simulink model "x220KVSSTN_slx"  (R2025a)
settings: Solver=VariableStepAuto  StartTime=0.0  StopTime=1  RelTol=1e-4
libraries: spsThreePhaseSeriesRLCLoadLib x16, spsThreePhasePISectionLineLib x15, spsThreePhaseBreakerLib x8, spsThreePhaseVIMeasurementLib x7, spsThreePhaseTransformerTwoWindingsLib x5, spsLoadFlowBusLib x4, spsThreePhaseSourceLib x3, spsRMSLib x1, spsThreePhaseFaultLib x1, sps_lib x1
settings Model: Creator=ARYAN CHOUDHARY  LastModifiedBy=ARYAN CHOUDHARY

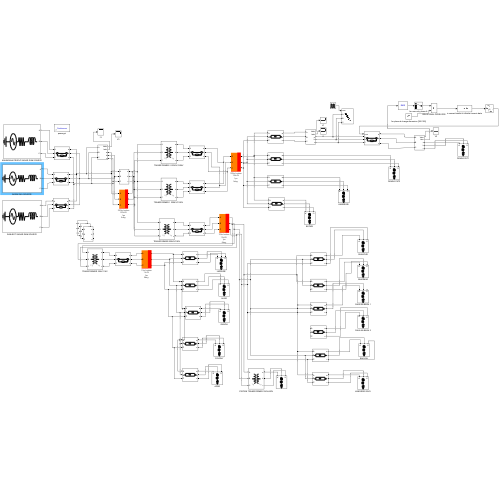
[thumbnail: Simulink's stored preview of the top-level diagram]
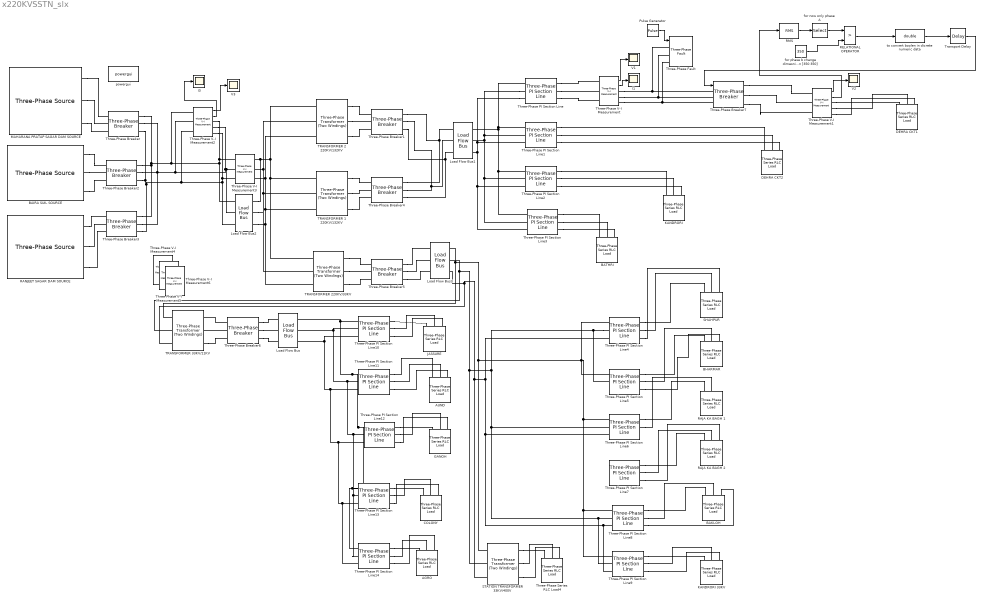
== system x220KVSSTN_slx ==
  AGRO : spsThreePhaseSeriesRLCLoadLib/Three-Phase Series RLC Load  LConnTagsString=A|B|C  Configuration=Y (grounded)  NominalVoltage=132e3  Vabc=[1e3 1e3 1e3]  Vabcp=[1e3 1e3 1e3]  NominalFrequency=50  UnbalancedPower=off  ActivePower=50e6  InductivePower=10e6  CapacitivePower=10e6  Pabc=[10e3 9e3 11e3]  QLabc=[100 90 110]  QCabc=[100 90 110]  Pabcp=[10e3 9e3 11e3]  QLabcp=[100 90 110]  QCabcp=[100 90 110]  Measurements=None  LoadType=constant PQ
  AUND : spsThreePhaseSeriesRLCLoadLib/Three-Phase Series RLC Load  LConnTagsString=A|B|C  Configuration=Y (grounded)  NominalVoltage=132e3  Vabc=[1e3 1e3 1e3]  Vabcp=[1e3 1e3 1e3]  NominalFrequency=50  UnbalancedPower=off  ActivePower=50e6  InductivePower=10e6  CapacitivePower=10e6  Pabc=[10e3 9e3 11e3]  QLabc=[100 90 110]  QCabc=[100 90 110]  Pabcp=[10e3 9e3 11e3]  QLabcp=[100 90 110]  QCabcp=[100 90 110]  Measurements=None  LoadType=constant PQ
  BAIRA SUIL SOURCE : spsThreePhaseSourceLib/Three-Phase Source  InternalConnection=Yg  VoltagePhases=off  Voltage=220e3  PhaseAngle=0  Voltage_phases=[25e3 25e3 25e3]/sqrt(3)  PhaseAngles_phases=[0 -120 +120]  Frequency=50  NonIdealSource=on  SpecifyImpedance=off  Resistance=0.8929  Inductance=16.58e-3  ShortCircuitLevel=100e6  BaseVoltage=25e3  XRratio=7  BusType=PQ  Pref=50e6  Qref=10e6  Prefabc=[10e3, 10e3, 10e3]  Qrefabc=[0, 0, 0]  Qmin=-inf  Qmax=inf
  BAKLOH : spsThreePhaseSeriesRLCLoadLib/Three-Phase Series RLC Load  LConnTagsString=A|B|C  Configuration=Y (grounded)  NominalVoltage=132e3  Vabc=[1e3 1e3 1e3]  Vabcp=[1e3 1e3 1e3]  NominalFrequency=50  UnbalancedPower=off  ActivePower=50e6  InductivePower=10e6  CapacitivePower=10e6  Pabc=[10e3 9e3 11e3]  QLabc=[100 90 110]  QCabc=[100 90 110]  Pabcp=[10e3 9e3 11e3]  QLabcp=[100 90 110]  QCabcp=[100 90 110]  Measurements=None  LoadType=constant PQ
  BATHRI : spsThreePhaseSeriesRLCLoadLib/Three-Phase Series RLC Load  LConnTagsString=A|B|C  Configuration=Y (grounded)  NominalVoltage=132e3  Vabc=[1e3 1e3 1e3]  Vabcp=[1e3 1e3 1e3]  NominalFrequency=50  UnbalancedPower=off  ActivePower=50e6  InductivePower=10e6  CapacitivePower=10e6  Pabc=[10e3 9e3 11e3]  QLabc=[100 90 110]  QCabc=[100 90 110]  Pabcp=[10e3 9e3 11e3]  QLabcp=[100 90 110]  QCabcp=[100 90 110]  Measurements=None  LoadType=constant PQ
  BHARMAR : spsThreePhaseSeriesRLCLoadLib/Three-Phase Series RLC Load  LConnTagsString=A|B|C  Configuration=Y (grounded)  NominalVoltage=132e3  Vabc=[1e3 1e3 1e3]  Vabcp=[1e3 1e3 1e3]  NominalFrequency=50  UnbalancedPower=off  ActivePower=50e6  InductivePower=10e6  CapacitivePower=10e6  Pabc=[10e3 9e3 11e3]  QLabc=[100 90 110]  QCabc=[100 90 110]  Pabcp=[10e3 9e3 11e3]  QLabcp=[100 90 110]  QCabcp=[100 90 110]  Measurements=None  LoadType=constant PQ
  COLONY : spsThreePhaseSeriesRLCLoadLib/Three-Phase Series RLC Load  LConnTagsString=A|B|C  Configuration=Y (grounded)  NominalVoltage=132e3  Vabc=[1e3 1e3 1e3]  Vabcp=[1e3 1e3 1e3]  NominalFrequency=50  UnbalancedPower=off  ActivePower=50e6  InductivePower=10e6  CapacitivePower=10e6  Pabc=[10e3 9e3 11e3]  QLabc=[100 90 110]  QCabc=[100 90 110]  Pabcp=[10e3 9e3 11e3]  QLabcp=[100 90 110]  QCabcp=[100 90 110]  Measurements=None  LoadType=constant PQ
  DEHRA CKT1 : spsThreePhaseSeriesRLCLoadLib/Three-Phase Series RLC Load  LConnTagsString=A|B|C  Configuration=Y (grounded)  NominalVoltage=132e3  Vabc=[1e3 1e3 1e3]  Vabcp=[1e3 1e3 1e3]  NominalFrequency=50  UnbalancedPower=off  ActivePower=50e6  InductivePower=10e6  CapacitivePower=10e6  Pabc=[10e3 9e3 11e3]  QLabc=[100 90 110]  QCabc=[100 90 110]  Pabcp=[10e3 9e3 11e3]  QLabcp=[100 90 110]  QCabcp=[100 90 110]  Measurements=None  LoadType=constant PQ
  DEHRA CKT2 : spsThreePhaseSeriesRLCLoadLib/Three-Phase Series RLC Load  LConnTagsString=A|B|C  Configuration=Y (grounded)  NominalVoltage=132e3  Vabc=[1e3 1e3 1e3]  Vabcp=[1e3 1e3 1e3]  NominalFrequency=50  UnbalancedPower=off  ActivePower=50e6  InductivePower=10e6  CapacitivePower=10e6  Pabc=[10e3 9e3 11e3]  QLabc=[100 90 110]  QCabc=[100 90 110]  Pabcp=[10e3 9e3 11e3]  QLabcp=[100 90 110]  QCabcp=[100 90 110]  Measurements=None  LoadType=constant PQ
  GANOH : spsThreePhaseSeriesRLCLoadLib/Three-Phase Series RLC Load  LConnTagsString=A|B|C  Configuration=Y (grounded)  NominalVoltage=132e3  Vabc=[1e3 1e3 1e3]  Vabcp=[1e3 1e3 1e3]  NominalFrequency=50  UnbalancedPower=off  ActivePower=50e6  InductivePower=10e6  CapacitivePower=10e6  Pabc=[10e3 9e3 11e3]  QLabc=[100 90 110]  QCabc=[100 90 110]  Pabcp=[10e3 9e3 11e3]  QLabcp=[100 90 110]  QCabcp=[100 90 110]  Measurements=None  LoadType=constant PQ
  I1 : Scope
      settings: ActiveDisplayYMinimum=-9501.2385556277131  ActiveDisplayYMaximum=13987.721223834153
  I3 : Scope
      settings: ActiveDisplayYMinimum=-31.371418582572904  ActiveDisplayYMaximum=38.377449294151894  DataLoggingVariableName=ScopeData4
  JASSURE : spsThreePhaseSeriesRLCLoadLib/Three-Phase Series RLC Load  LConnTagsString=A|B|C  Configuration=Y (grounded)  NominalVoltage=132e3  Vabc=[1e3 1e3 1e3]  Vabcp=[1e3 1e3 1e3]  NominalFrequency=50  UnbalancedPower=off  ActivePower=50e6  InductivePower=10e6  CapacitivePower=10e6  Pabc=[10e3 9e3 11e3]  QLabc=[100 90 110]  QCabc=[100 90 110]  Pabcp=[10e3 9e3 11e3]  QLabcp=[100 90 110]  QCabcp=[100 90 110]  Measurements=None  LoadType=constant PQ
  KANDRORI : spsThreePhaseSeriesRLCLoadLib/Three-Phase Series RLC Load  LConnTagsString=A|B|C  Configuration=Y (grounded)  NominalVoltage=132e3  Vabc=[1e3 1e3 1e3]  Vabcp=[1e3 1e3 1e3]  NominalFrequency=50  UnbalancedPower=off  ActivePower=50e6  InductivePower=10e6  CapacitivePower=10e6  Pabc=[10e3 9e3 11e3]  QLabc=[100 90 110]  QCabc=[100 90 110]  Pabcp=[10e3 9e3 11e3]  QLabcp=[100 90 110]  QCabcp=[100 90 110]  Measurements=None  LoadType=constant PQ
  KANDRORI 33KV : spsThreePhaseSeriesRLCLoadLib/Three-Phase Series RLC Load  LConnTagsString=A|B|C  Configuration=Y (grounded)  NominalVoltage=132e3  Vabc=[1e3 1e3 1e3]  Vabcp=[1e3 1e3 1e3]  NominalFrequency=50  UnbalancedPower=off  ActivePower=50e6  InductivePower=10e6  CapacitivePower=10e6  Pabc=[10e3 9e3 11e3]  QLabc=[100 90 110]  QCabc=[100 90 110]  Pabcp=[10e3 9e3 11e3]  QLabcp=[100 90 110]  QCabcp=[100 90 110]  Measurements=None  LoadType=constant PQ
  Load Flow Bus : spsLoadFlowBusLib/Load Flow Bus  LConnTagsString=a|b|c  RConnTagsString=a|b|c  Phases=ABC  Connectors=on both sides  ID=11kv busbar  Vbase=11e3  Vref=[1 1 1]  Vangle=[0 0 0]  VLF=1  VLFb=1  VLFc=1  angleLF=0  angleLFb=0  angleLFc=0
  Load Flow Bus1 : spsLoadFlowBusLib/Load Flow Bus  LConnTagsString=a|b|c  RConnTagsString=a|b|c  Phases=ABC  Connectors=on both sides  ID=132kv busbar  Vbase=132e3  Vref=[1 1 1]  Vangle=[0 0 0]  VLF=1  VLFb=1  VLFc=1  angleLF=0  angleLFb=0  angleLFc=0
  Load Flow Bus2 : spsLoadFlowBusLib/Load Flow Bus  LConnTagsString=a|b|c  RConnTagsString=a|b|c  Phases=ABC  Connectors=on both sides  ID=220kv busbar  Vbase=220e3  Vref=[1 1 1]  Vangle=[0 0 0]  VLF=1  VLFb=1  VLFc=1  angleLF=0  angleLFb=0  angleLFc=0
  Load Flow Bus3 : spsLoadFlowBusLib/Load Flow Bus  LConnTagsString=a|b|c  RConnTagsString=a|b|c  Phases=ABC  Connectors=on both sides  ID=33kv busbar  Vbase=33e3  Vref=[1 1 1]  Vangle=[0 0 0]  VLF=1  VLFb=1  VLFc=1  angleLF=0  angleLFb=0  angleLFc=0
  MAHARANA PRATAP SAGAR DAM SOURCE : spsThreePhaseSourceLib/Three-Phase Source  InternalConnection=Yg  VoltagePhases=off  Voltage=220e3  PhaseAngle=0  Voltage_phases=[25e3 25e3 25e3]/sqrt(3)  PhaseAngles_phases=[0 -120 +120]  Frequency=50  NonIdealSource=on  SpecifyImpedance=off  Resistance=0.8929  Inductance=16.58e-3  ShortCircuitLevel=100e6  BaseVoltage=25e3  XRratio=7  BusType=swing  Pref=10e3  Qref=0  Prefabc=[10e3, 10e3, 10e3]  Qrefabc=[0, 0, 0]  Qmin=-inf  Qmax=inf
  Pulse Generator : DiscretePulseGenerator  PulseType=Time based  Period=10  PhaseDelay=0.2
  RAJA KA BAGH 1 : spsThreePhaseSeriesRLCLoadLib/Three-Phase Series RLC Load  LConnTagsString=A|B|C  Configuration=Y (grounded)  NominalVoltage=132e3  Vabc=[1e3 1e3 1e3]  Vabcp=[1e3 1e3 1e3]  NominalFrequency=50  UnbalancedPower=off  ActivePower=50e6  InductivePower=10e6  CapacitivePower=10e6  Pabc=[10e3 9e3 11e3]  QLabc=[100 90 110]  QCabc=[100 90 110]  Pabcp=[10e3 9e3 11e3]  QLabcp=[100 90 110]  QCabcp=[100 90 110]  Measurements=None  LoadType=constant PQ
  RAJA KA BAGH 2 : spsThreePhaseSeriesRLCLoadLib/Three-Phase Series RLC Load  LConnTagsString=A|B|C  Configuration=Y (grounded)  NominalVoltage=132e3  Vabc=[1e3 1e3 1e3]  Vabcp=[1e3 1e3 1e3]  NominalFrequency=50  UnbalancedPower=off  ActivePower=50e6  InductivePower=10e6  CapacitivePower=10e6  Pabc=[10e3 9e3 11e3]  QLabc=[100 90 110]  QCabc=[100 90 110]  Pabcp=[10e3 9e3 11e3]  QLabcp=[100 90 110]  QCabcp=[100 90 110]  Measurements=None  LoadType=constant PQ
  RANJEET SAGAR DAM SOURCE : spsThreePhaseSourceLib/Three-Phase Source  InternalConnection=Yg  VoltagePhases=off  Voltage=220e3  PhaseAngle=0  Voltage_phases=[25e3 25e3 25e3]/sqrt(3)  PhaseAngles_phases=[0 -120 +120]  Frequency=50  NonIdealSource=on  SpecifyImpedance=off  Resistance=0.8929  Inductance=16.58e-3  ShortCircuitLevel=100e6  BaseVoltage=25e3  XRratio=7  BusType=PQ  Pref=50e6  Qref=10e6  Prefabc=[10e3, 10e3, 10e3]  Qrefabc=[0, 0, 0]  Qmin=-inf  Qmax=inf
  RELATIONAL OPERATOR : RelationalOperator  Operator=>  OutDataTypeStr=boolean  RndMeth=Simplest  InputSameDT=off
  RMS : spsRMSLib/RMS  TrueRMS=on  Freq=50  RMSInit=341  Ts=0
  SHAHPUR : spsThreePhaseSeriesRLCLoadLib/Three-Phase Series RLC Load  LConnTagsString=A|B|C  Configuration=Y (grounded)  NominalVoltage=132e3  Vabc=[1e3 1e3 1e3]  Vabcp=[1e3 1e3 1e3]  NominalFrequency=50  UnbalancedPower=off  ActivePower=50e6  InductivePower=10e6  CapacitivePower=10e6  Pabc=[10e3 9e3 11e3]  QLabc=[100 90 110]  QCabc=[100 90 110]  Pabcp=[10e3 9e3 11e3]  QLabcp=[100 90 110]  QCabcp=[100 90 110]  Measurements=None  LoadType=constant PQ
  STATION TRANSFORMER 33KV/400V : spsThreePhaseTransformerTwoWindingsLib/Three-Phase Transformer (Two Windings)  Winding1Connection=Yg  Winding2Connection=Yg  CoreType=Three single-phase transformers  SetSaturation=off  Hysteresis=off  DataFile='hysteresis'  SetInitialFlux=off  Measurements=None  UNITS=pu  NominalPower=[ 400e3 , 50 ]  Winding1=[33e3 , 0.002 , 0.08 ]  Winding2=[4e2 , 0.002 , 0.08 ]  Rm=500  Lm=500  L0=0.5  Saturation=[ 0,0 ; 0.0024,1.2 ; 1.0,1.52 ]  InitialFluxes=[ 0.8 , -0.8 , 0.7 ]  BreakLoop=off  DiscreteSolver=Trapezoidal iterative  DataType=off  TransfoNumber=1
  "TRANSFORMER 1 220KV/132KV " : spsThreePhaseTransformerTwoWindingsLib/Three-Phase Transformer (Two Windings)  Winding1Connection=Yg  Winding2Connection=Yg  CoreType=Three single-phase transformers  SetSaturation=off  Hysteresis=off  DataFile='hysteresis'  SetInitialFlux=off  Measurements=None  UNITS=pu  NominalPower=[ 63e6 , 50 ]  Winding1=[ 220e3 , 0.002 , 0.08 ]  Winding2=[ 132e3 , 0.002 , 0.08 ]  Rm=500  Lm=500  L0=0.5  Saturation=[ 0,0 ; 0.0024,1.2 ; 1.0,1.52 ]  InitialFluxes=[ 0.8 , -0.8 , 0.7 ]  BreakLoop=off  DiscreteSolver=Trapezoidal iterative  DataType=off  TransfoNumber=1
  TRANSFORMER 2 220KV/132KV : spsThreePhaseTransformerTwoWindingsLib/Three-Phase Transformer (Two Windings)  Winding1Connection=Yg  Winding2Connection=Yg  CoreType=Three single-phase transformers  SetSaturation=off  Hysteresis=off  DataFile='hysteresis'  SetInitialFlux=off  Measurements=None  UNITS=pu  NominalPower=[ 150e6 , 50 ]  Winding1=[ 220e3 , 0.002 , 0.08 ]  Winding2=[ 132e3 , 0.002 , 0.08 ]  Rm=500  Lm=500  L0=0.5  Saturation=[ 0,0 ; 0.0024,1.2 ; 1.0,1.52 ]  InitialFluxes=[ 0.8 , -0.8 , 0.7 ]  BreakLoop=off  DiscreteSolver=Trapezoidal iterative  DataType=off  TransfoNumber=1
  TRANSFORMER 220KV/33KV : spsThreePhaseTransformerTwoWindingsLib/Three-Phase Transformer (Two Windings)  Winding1Connection=Yg  Winding2Connection=Yg  CoreType=Three single-phase transformers  SetSaturation=off  Hysteresis=off  DataFile='hysteresis'  SetInitialFlux=off  Measurements=None  UNITS=pu  NominalPower=[ 31.5e6 , 50 ]  Winding1=[ 220e3 , 0.002 , 0.08 ]  Winding2=[33e3 , 0.002 , 0.08 ]  Rm=500  Lm=500  L0=0.5  Saturation=[ 0,0 ; 0.0024,1.2 ; 1.0,1.52 ]  InitialFluxes=[ 0.8 , -0.8 , 0.7 ]  BreakLoop=off  DiscreteSolver=Trapezoidal iterative  DataType=off  TransfoNumber=1
  TRANSFORMER 33KV/11KV : spsThreePhaseTransformerTwoWindingsLib/Three-Phase Transformer (Two Windings)  Winding1Connection=Yg  Winding2Connection=Yg  CoreType=Three single-phase transformers  SetSaturation=off  Hysteresis=off  DataFile='hysteresis'  SetInitialFlux=off  Measurements=None  UNITS=pu  NominalPower=[ 10e6 , 50 ]  Winding1=[33e3 , 0.002 , 0.08 ]  Winding2=[11e3 , 0.002 , 0.08 ]  Rm=500  Lm=500  L0=0.5  Saturation=[ 0,0 ; 0.0024,1.2 ; 1.0,1.52 ]  InitialFluxes=[ 0.8 , -0.8 , 0.7 ]  BreakLoop=off  DiscreteSolver=Trapezoidal iterative  DataType=off  TransfoNumber=1
  Three-Phase PI Section Line : spsThreePhasePISectionLineLib/Three-Phase PI Section Line  LConnTagsString=a|b|c  RConnTagsString=A|B|C  Length=34  Frequency=50  Resistances=[ 0.01273 0.3864]  Inductances="[ 0.9337e-3  4.1264e-3]"  Capacitances=[12.74e-9 7.751e-9]
  Three-Phase PI Section Line{1..14} (14 alike) : spsThreePhasePISectionLineLib/Three-Phase PI Section Line  LConnTagsString=a|b|c  RConnTagsString=A|B|C  Length=100  Frequency=50  Resistances=[ 0.01273 0.3864]  Inductances="[ 0.9337e-3  4.1264e-3]"  Capacitances=[12.74e-9 7.751e-9]
  Three-Phase Series RLC Load4 : spsThreePhaseSeriesRLCLoadLib/Three-Phase Series RLC Load  LConnTagsString=A|B|C  Configuration=Y (grounded)  NominalVoltage=132e3  Vabc=[1e3 1e3 1e3]  Vabcp=[1e3 1e3 1e3]  NominalFrequency=50  UnbalancedPower=off  ActivePower=320e3  InductivePower=200e3  CapacitivePower=50e3  Pabc=[10e3 9e3 11e3]  QLabc=[100 90 110]  QCabc=[100 90 110]  Pabcp=[10e3 9e3 11e3]  QLabcp=[100 90 110]  QCabcp=[100 90 110]  Measurements=None  LoadType=constant Z
  Three-Phase V-I Measurement : spsThreePhaseVIMeasurementLib/Three-Phase V-I Measurement  VoltageMeasurement=phase-to-ground  SetLabelV=off  LabelV=Vabc  Vpu=off  VpuLL=off  CurrentMeasurement=yes  SetLabelI=off  LabelI=Iabc  Ipu=off  Pbase=100e6  Vbase=500e3  OutputType=Complex  PhasorSimulation=off  PSBequivalent=0
  Three-Phase V-I Measurement1 : spsThreePhaseVIMeasurementLib/Three-Phase V-I Measurement  VoltageMeasurement=phase-to-ground  SetLabelV=off  LabelV=Vabc  Vpu=off  VpuLL=off  CurrentMeasurement=yes  SetLabelI=off  LabelI=Iabc  Ipu=off  Pbase=100e6  Vbase=500e3  OutputType=Complex  PhasorSimulation=off  PSBequivalent=0
  Three-Phase V-I Measurement2 : spsThreePhaseVIMeasurementLib/Three-Phase V-I Measurement  VoltageMeasurement=phase-to-ground  SetLabelV=off  LabelV=Vabc  Vpu=off  VpuLL=off  CurrentMeasurement=yes  SetLabelI=off  LabelI=Iabc  Ipu=off  Pbase=100e6  Vbase=500e3  OutputType=Complex  PhasorSimulation=off  PSBequivalent=0
  Three-Phase V-I Measurement{3..6} (4 alike) : spsThreePhaseVIMeasurementLib/Three-Phase V-I Measurement  VoltageMeasurement=no  SetLabelV=off  LabelV=Vabc  Vpu=off  VpuLL=off  CurrentMeasurement=no  SetLabelI=off  LabelI=Iabc  Ipu=off  Pbase=100e6  Vbase=500e3  OutputType=Complex  PhasorSimulation=off  PSBequivalent=0
  Three-Phase Breaker{,1..6} (7 alike) : spsThreePhaseBreakerLib/Three-Phase Breaker  InitialState=closed  SwitchA=on  SwitchB=on  SwitchC=on  SwitchTimes="[1/60  5/60]"  External=off  BreakerResistance=0.11  SnubberResistance=1e6  SnubberCapacitance=inf  Measurements=None
  Three-Phase Breaker7 : spsThreePhaseBreakerLib/Three-Phase Breaker  InitialState=closed  SwitchA=on  SwitchB=on  SwitchC=on  SwitchTimes="[1/60  5/60]"  External=on  BreakerResistance=0.11  SnubberResistance=1e6  SnubberCapacitance=inf  Measurements=None
  Three-Phase Fault : spsThreePhaseFaultLib/Three-Phase Fault  InitialStates=0  FaultA=on  FaultB=off  FaultC=off  GroundFault=on  SwitchTimes="[1/60  5/60]"  External=on  SwitchStatus=NaN  FaultResistance=0.01  GroundResistance=0.01  SnubberResistance=1e6  SnubberCapacitance=inf  Measurements=None
  Transport Delay : TransportDelay  DelayTime=0.2  BufferSize=30720
  V1 : Scope
      settings: ActiveDisplayYMinimum=-134175.28868127437  ActiveDisplayYMaximum=134108.09321994495
  V2 : Scope
      settings: ActiveDisplayYMinimum=-26718.305240557729  ActiveDisplayYMaximum=43984.791474851641  DataLoggingVariableName=ScopeData2
  V3 : Scope
      settings: ActiveDisplayYMinimum=-102465.81313536782  ActiveDisplayYMaximum=252772.60043735284  DataLoggingVariableName=ScopeData5
  for now only phase A : Selector  InputPortWidth=3  IndexOptions=Index vector (dialog)  Indices=1  OutputSizes=1
  for phase b change dimesnion [350 350] : Constant  Value=350  VectorParams1D=off
  powergui : sps_lib/powergui  Priority=1  SimulationMode=Continuous  SampleTime=50e-6  frequency=50  Iterations=50  frequencyindice=50  Pbase=100e6  ErrMax=1e-4  UnitsV=kV  UnitsW=MW  buscounter=0  FunctionMessages=off  echomessages=off  EnableUseOfTLC=off  CurrentSourceSwitches=off  DisableSnubberDevices=off  DisableRonSwitches=off  DisableVfSwitches=off  DisplayEquations=off  AutomaticDiscreteSolvers=off  SolverType=Tustin/Backward Euler (TBE)  Interpol=off  ExternalGateDelay=off  methode=off  Ts=100  x0status=blocks  SPID=on  SwTol=0  HookPort=off  NonlinearTolerance=1e-4  nMaxIteration=100  ContinueOnMaxIteration=off  RestoreLinks=warning  ResistiveCurrentMeasurement=off  Frange=[0:2:500]  Ylog=off  Xlog=on  ShowGrid=off  save=off  variable=ZData  structure=0  ZoomFFT=off  StartTime=0.0  cycles=1  DisplayStyle=1  fundamental=60  FreqAxis=off  MaxFrequency=1000  frequencyindicesteady=1  RmsSteady=1  display=off
  "to convert boolen in dicrete numeric data " : DataTypeConversion  OutDataTypeStr=double  SaturateOnIntegerOverflow=off  RndMeth=Floor
  wires:
  Three-Phase V-I Measurement/1 -> V1/1
  Three-Phase V-I Measurement/2 -> I1/1
  Three-Phase V-I Measurement1/1 -> V2/1
  Three-Phase V-I Measurement1/2 -> RMS/1
  Three-Phase V-I Measurement2/1 -> V3/1
  Three-Phase V-I Measurement2/2 -> I3/1
  Pulse Generator/1 -> Three-Phase Fault/1
  RELATIONAL OPERATOR/1 -> "to convert boolen in dicrete numeric data "/1
  Transport Delay/1 -> Three-Phase Breaker7/1
  RMS/1 -> for now only phase A/1
  for now only phase A/1 -> RELATIONAL OPERATOR/1
  for phase b change dimesnion [350 350]/1 -> RELATIONAL OPERATOR/2
  "to convert boolen in dicrete numeric data "/1 -> Transport Delay/1
  connections:
  MAHARANA PRATAP SAGAR DAM SOURCE/RConn1 -- Three-Phase Breaker/LConn1
  MAHARANA PRATAP SAGAR DAM SOURCE/RConn2 -- Three-Phase Breaker/LConn2
  MAHARANA PRATAP SAGAR DAM SOURCE/RConn3 -- Three-Phase Breaker/LConn3
  TRANSFORMER 2 220KV/132KV/RConn1 -- Three-Phase Breaker1/LConn1
  TRANSFORMER 2 220KV/132KV/RConn2 -- Three-Phase Breaker1/LConn2
  TRANSFORMER 2 220KV/132KV/RConn3 -- Three-Phase Breaker1/LConn3
  BAIRA SUIL SOURCE/RConn1 -- Three-Phase Breaker2/LConn1
  BAIRA SUIL SOURCE/RConn2 -- Three-Phase Breaker2/LConn2
  BAIRA SUIL SOURCE/RConn3 -- Three-Phase Breaker2/LConn3
  RANJEET SAGAR DAM SOURCE/RConn1 -- Three-Phase Breaker3/LConn1
  RANJEET SAGAR DAM SOURCE/RConn2 -- Three-Phase Breaker3/LConn2
  RANJEET SAGAR DAM SOURCE/RConn3 -- Three-Phase Breaker3/LConn3
  Three-Phase Breaker/RConn1 -- Three-Phase Breaker3/RConn1 -- Three-Phase Breaker2/RConn1 -- Three-Phase V-I Measurement2/LConn1 -- Three-Phase V-I Measurement3/LConn1 -- Three-Phase V-I Measurement2/RConn1 -- Load Flow Bus2/LConn1
  Three-Phase Breaker2/RConn2 -- Three-Phase Breaker3/RConn2 -- Three-Phase Breaker/RConn2 -- Three-Phase V-I Measurement2/LConn2 -- Load Flow Bus2/LConn2 -- Three-Phase V-I Measurement3/LConn2 -- Three-Phase V-I Measurement2/RConn2
  Three-Phase Breaker/RConn3 -- Three-Phase Breaker3/RConn3 -- Three-Phase V-I Measurement2/LConn3 -- Load Flow Bus2/LConn3 -- Three-Phase V-I Measurement2/RConn3 -- Three-Phase V-I Measurement3/LConn3 -- Three-Phase Breaker2/RConn3
  TRANSFORMER 220KV/33KV/LConn1 -- "TRANSFORMER 1 220KV/132KV "/LConn1 -- TRANSFORMER 2 220KV/132KV/LConn1 -- Load Flow Bus2/RConn1 -- Three-Phase V-I Measurement3/RConn1
  "TRANSFORMER 1 220KV/132KV "/LConn2 -- TRANSFORMER 220KV/33KV/LConn2 -- Load Flow Bus2/RConn2 -- Three-Phase V-I Measurement3/RConn2 -- TRANSFORMER 2 220KV/132KV/LConn2
  "TRANSFORMER 1 220KV/132KV "/LConn3 -- Load Flow Bus2/RConn3 -- TRANSFORMER 220KV/33KV/LConn3 -- Three-Phase V-I Measurement3/RConn3 -- TRANSFORMER 2 220KV/132KV/LConn3
  "TRANSFORMER 1 220KV/132KV "/RConn1 -- Three-Phase Breaker4/LConn1
  "TRANSFORMER 1 220KV/132KV "/RConn2 -- Three-Phase Breaker4/LConn2
  "TRANSFORMER 1 220KV/132KV "/RConn3 -- Three-Phase Breaker4/LConn3
  Three-Phase Breaker1/RConn1 -- Three-Phase Breaker4/RConn1 -- Load Flow Bus1/LConn1
  Three-Phase Breaker1/RConn2 -- Three-Phase Breaker4/RConn2 -- Load Flow Bus1/LConn2
  Three-Phase Breaker1/RConn3 -- Three-Phase Breaker4/RConn3 -- Load Flow Bus1/LConn3
  TRANSFORMER 220KV/33KV/RConn1 -- Three-Phase Breaker5/LConn1
  TRANSFORMER 220KV/33KV/RConn2 -- Three-Phase Breaker5/LConn2
  TRANSFORMER 220KV/33KV/RConn3 -- Three-Phase Breaker5/LConn3
  Three-Phase Breaker5/RConn1 -- Load Flow Bus3/LConn1
  Three-Phase Breaker5/RConn2 -- Load Flow Bus3/LConn2
  Three-Phase Breaker5/RConn3 -- Load Flow Bus3/LConn3
  Three-Phase PI Section Line/LConn1 -- Three-Phase PI Section Line3/LConn1 -- Three-Phase PI Section Line2/LConn1 -- Load Flow Bus1/RConn1 -- Three-Phase PI Section Line1/LConn1
  Three-Phase PI Section Line/LConn2 -- Three-Phase PI Section Line3/LConn2 -- Three-Phase PI Section Line2/LConn2 -- Load Flow Bus1/RConn2 -- Three-Phase PI Section Line1/LConn2
  Three-Phase PI Section Line/LConn3 -- Three-Phase PI Section Line3/LConn3 -- Three-Phase PI Section Line2/LConn3 -- Load Flow Bus1/RConn3 -- Three-Phase PI Section Line1/LConn3
  Three-Phase Fault/LConn1 -- Three-Phase V-I Measurement/RConn1 -- Three-Phase Breaker7/LConn1
  Three-Phase Fault/LConn2 -- Three-Phase V-I Measurement/RConn2 -- Three-Phase Breaker7/LConn2
  Three-Phase Fault/LConn3 -- Three-Phase V-I Measurement/RConn3 -- Three-Phase Breaker7/LConn3
  Three-Phase PI Section Line1/RConn1 -- DEHRA CKT2/LConn1
  Three-Phase PI Section Line1/RConn2 -- DEHRA CKT2/LConn2
  Three-Phase PI Section Line1/RConn3 -- DEHRA CKT2/LConn3
  Three-Phase PI Section Line2/RConn1 -- KANDRORI/LConn1
  Three-Phase PI Section Line2/RConn2 -- KANDRORI/LConn2
  Three-Phase PI Section Line2/RConn3 -- KANDRORI/LConn3
  Three-Phase PI Section Line3/RConn1 -- BATHRI/LConn1
  Three-Phase PI Section Line3/RConn2 -- BATHRI/LConn2
  Three-Phase PI Section Line3/RConn3 -- BATHRI/LConn3
  Three-Phase PI Section Line4/RConn1 -- SHAHPUR/LConn1
  Three-Phase PI Section Line4/RConn2 -- SHAHPUR/LConn2
  Three-Phase PI Section Line4/RConn3 -- SHAHPUR/LConn3
  Three-Phase PI Section Line5/RConn1 -- BHARMAR/LConn1
  Three-Phase PI Section Line5/RConn2 -- BHARMAR/LConn2
  Three-Phase PI Section Line5/RConn3 -- BHARMAR/LConn3
  Three-Phase PI Section Line6/RConn1 -- RAJA KA BAGH 1/LConn1
  Three-Phase PI Section Line6/RConn2 -- RAJA KA BAGH 1/LConn2
  Three-Phase PI Section Line7/RConn1 -- RAJA KA BAGH 2/LConn1
  Three-Phase PI Section Line7/RConn2 -- RAJA KA BAGH 2/LConn2
  Three-Phase PI Section Line7/RConn3 -- RAJA KA BAGH 2/LConn3
  Three-Phase PI Section Line8/RConn1 -- BAKLOH/LConn1
  Three-Phase PI Section Line8/RConn2 -- BAKLOH/LConn2
  Three-Phase PI Section Line8/RConn3 -- BAKLOH/LConn3
  Three-Phase PI Section Line9/RConn1 -- KANDRORI 33KV/LConn1
  Three-Phase PI Section Line9/RConn2 -- KANDRORI 33KV/LConn2
  Three-Phase PI Section Line9/RConn3 -- KANDRORI 33KV/LConn3
  Three-Phase PI Section Line4/LConn2 -- Load Flow Bus3/RConn2 -- TRANSFORMER 33KV/11KV/LConn2 -- STATION TRANSFORMER 33KV/400V/LConn2 -- Three-Phase PI Section Line8/LConn2 -- Three-Phase PI Section Line9/LConn2 -- Three-Phase PI Section Line6/LConn2 -- Three-Phase PI Section Line5/LConn2
  Three-Phase PI Section Line9/LConn3 -- Three-Phase PI Section Line6/LConn3 -- TRANSFORMER 33KV/11KV/LConn3 -- Load Flow Bus3/RConn3 -- STATION TRANSFORMER 33KV/400V/LConn3 -- Three-Phase PI Section Line4/LConn3 -- Three-Phase PI Section Line8/LConn3
  Three-Phase PI Section Line5/LConn1 -- Load Flow Bus3/RConn1 -- TRANSFORMER 33KV/11KV/LConn1 -- STATION TRANSFORMER 33KV/400V/LConn1 -- Three-Phase PI Section Line6/LConn1 -- Three-Phase PI Section Line9/LConn1 -- Three-Phase PI Section Line8/LConn1 -- Three-Phase PI Section Line4/LConn1
  STATION TRANSFORMER 33KV/400V/RConn1 -- Three-Phase Series RLC Load4/LConn1
  STATION TRANSFORMER 33KV/400V/RConn2 -- Three-Phase Series RLC Load4/LConn2
  STATION TRANSFORMER 33KV/400V/RConn3 -- Three-Phase Series RLC Load4/LConn3
  Three-Phase Breaker6/LConn1 -- TRANSFORMER 33KV/11KV/RConn1
  Three-Phase Breaker6/LConn2 -- TRANSFORMER 33KV/11KV/RConn2
  TRANSFORMER 33KV/11KV/RConn3 -- Three-Phase Breaker6/LConn3
  Three-Phase Breaker6/RConn1 -- Load Flow Bus/LConn1
  Three-Phase Breaker6/RConn2 -- Load Flow Bus/LConn2
  Three-Phase Breaker6/RConn3 -- Load Flow Bus/LConn3
  Three-Phase PI Section Line11/LConn1 -- Three-Phase PI Section Line14/LConn1 -- Three-Phase PI Section Line13/LConn1 -- Three-Phase PI Section Line12/LConn1 -- Three-Phase PI Section Line10/LConn1 -- Load Flow Bus/RConn1
  Three-Phase PI Section Line11/LConn2 -- Three-Phase PI Section Line14/LConn2 -- Three-Phase PI Section Line13/LConn2 -- Three-Phase PI Section Line12/LConn2 -- Three-Phase PI Section Line10/LConn2 -- Load Flow Bus/RConn2
  Three-Phase PI Section Line11/LConn3 -- Three-Phase PI Section Line13/LConn3 -- Three-Phase PI Section Line14/LConn3 -- Three-Phase PI Section Line12/LConn3 -- Three-Phase PI Section Line10/LConn3 -- Load Flow Bus/RConn3
  Three-Phase PI Section Line14/RConn1 -- AGRO/LConn1
  Three-Phase PI Section Line14/RConn2 -- AGRO/LConn2
  Three-Phase PI Section Line14/RConn3 -- AGRO/LConn3
  Three-Phase PI Section Line13/RConn1 -- COLONY/LConn1
  Three-Phase PI Section Line13/RConn2 -- COLONY/LConn2
  Three-Phase PI Section Line13/RConn3 -- COLONY/LConn3
  Three-Phase PI Section Line12/RConn1 -- GANOH/LConn1
  Three-Phase PI Section Line12/RConn2 -- GANOH/LConn2
  Three-Phase PI Section Line12/RConn3 -- GANOH/LConn3
  Three-Phase PI Section Line11/RConn1 -- AUND/LConn1
  Three-Phase PI Section Line11/RConn2 -- AUND/LConn2
  Three-Phase PI Section Line11/RConn3 -- AUND/LConn3
  Three-Phase PI Section Line10/RConn1 -- JASSURE/LConn1
  Three-Phase PI Section Line10/RConn2 -- JASSURE/LConn2
  Three-Phase PI Section Line10/RConn3 -- JASSURE/LConn3
  Three-Phase PI Section Line/RConn1 -- Three-Phase V-I Measurement/LConn1
  Three-Phase PI Section Line/RConn2 -- Three-Phase V-I Measurement/LConn2
  Three-Phase PI Section Line/RConn3 -- Three-Phase V-I Measurement/LConn3
  Three-Phase Breaker7/RConn1 -- Three-Phase V-I Measurement1/LConn1
  Three-Phase Breaker7/RConn2 -- Three-Phase V-I Measurement1/LConn2
  Three-Phase Breaker7/RConn3 -- Three-Phase V-I Measurement1/LConn3
  Three-Phase V-I Measurement1/RConn1 -- DEHRA CKT1/LConn1
  Three-Phase V-I Measurement1/RConn2 -- DEHRA CKT1/LConn2
  Three-Phase V-I Measurement1/RConn3 -- DEHRA CKT1/LConn3
